simulink model "FiveTwo_100"  (R2022b)
settings: Solver=VariableStepAuto  StartTime=0.0  StopTime=10.0  RelTol=1e-3
settings Model: Creator=yeyi5  LastModifiedBy=yeyi5

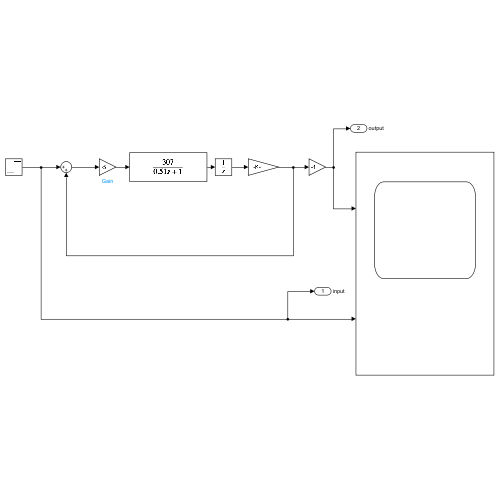
[thumbnail: Simulink's stored preview of the top-level diagram]
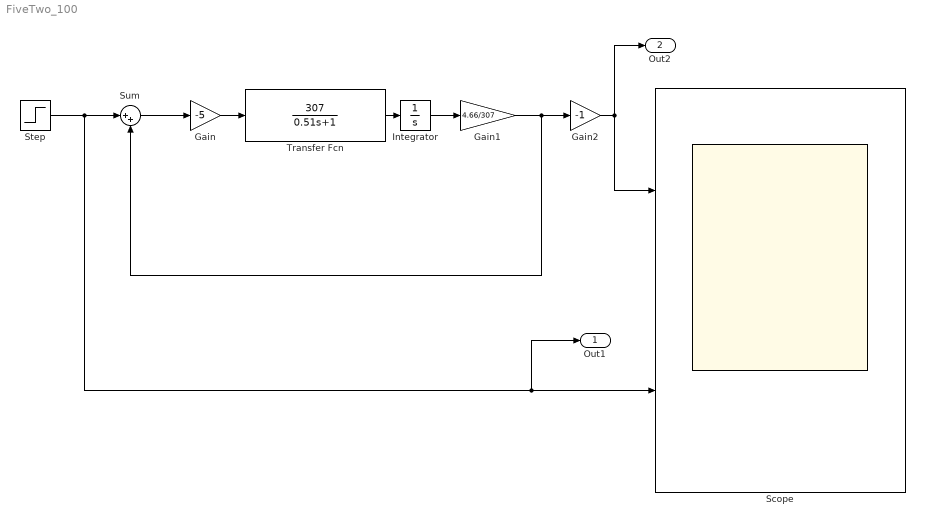
== system FiveTwo_100 ==
  Gain : Gain  Gain=-5
  Gain1 : Gain  Gain=4.66/307
  Gain2 : Gain  Gain=-1
  Integrator : Integrator
  Scope : Scope  NumInputPorts=2
  Step : Step  After=5  SampleTime=0
  Sum : Sum  Inputs=|++
  Transfer Fcn : TransferFcn  Numerator=[307]  Denominator=[0.51 1]
  Out1 : Outport  SignalName=input
  Out2 : Outport  Port=2  SignalName=output
  wires:
  Sum/1 -> Gain/1
  Transfer Fcn/1 -> Integrator/1
  Gain/1 -> Transfer Fcn/1
  Gain1/1 -> Sum/2, Gain2/1
  Integrator/1 -> Gain1/1
  Step/1 -> Out1/1, Scope/2, Sum/1
  Gain2/1 -> Out2/1, Scope/1
